simulink model "aircraftRamAirTurbineAssembly_MultiDomain"  (Simulink 7.9)
settings: Solver=ode23tb  StartTime=0.0  StopTime=6  FixedStep=Ts  MaxStep=50e-6  RelTol=1e-4
PreLoadFcn:
  | % PARAMETERS FOR HYDRAULIC CYLINDER
  | RO = 0.1;
  | t = 0.005;
  | h = 2.5;
  | lic = -1.1;
  | rho = 1000;
  | 
  | APist = pi*(RO - 2*t)*(RO - 2*t);
  | ROO = RO;
  | RIO = RO - t;
  | ROI = RO-t;
  | RII = RO- 2*t;
  | h_seg = h/2;
  | 
  | ro = ROO;
  | ri = RIO;
  | h = h_seg;
  | rho = rho;
  | rot_oc = [0 0 165];
  | 
  | mass_OC = rho*pi*(ro*ro-ri*ri)*h;
  | inertia_OC = mass_OC*([(3*ro*ro + h*h) 0 0;0 6*ro*ro 0;0 0 (3*ro*ro + h*h)]-[(3*ri*ri + h*h) 0 0;0 6*ri*ri 0;0 0 (3*ri*ri + h*h)])/12;
  | 
  | ro = ROI;
  | ri = RII;
  | h = h_seg;
  | rho = rho;
  | rot_ic = [0 0 0];
  | 
  | mass_IC = rho*pi*(ro*ro-ri*ri)*h;
  | inertia_IC = mass_IC*([(3*ro*ro + h*h) 0 0;0 6*ro*ro 0;0 0 (3*ro*ro + h*h)]-[(3*ri*ri + h*h) 0 0;0 6*ri*ri 0;0 0 (3*ri*ri + h*h)])/12;
  | 
  | a = 0.1;
  | b = 2;
  | c = 0.05;
  | rho = 1000;
  | theta = 180;
  | 
  | mass_Link = rho*a*b*c;
  | inertia_Link = rho*a*b*c*[(b^2+c^2) 0 0; 0 (a^2+c^2) 0; 0 0 (a^2+b^2)]/12;
  | 
  | Actuator_Attach_Pt = [0 -0.2 0];
  | Actuator_Wing_Pt = [-0.5 0 0];
  | Outer_Cylinder_Length = 0.35;
  | Inner_Cylinder_Length = 0.25;
  | 
  | Outer_Cyl_Axis = Actuator_Wing_Pt - Actuator_Attach_Pt;
  | %Outer_Cyl_Axis = Outer_Cyl_Axis/(sqrt(sum(Outer_Cyl_Axis.*Outer_Cyl_Axis)));
  | 
  | %Actuator_Angle = atan(Outer_Cyl_Axis(2)/Outer_Cyl_Axis(1))*180/pi;
  | Actuator_Angle = -10;
  | Outer_Cyl_CS2 = Outer_Cyl_Axis*Outer_Cylinder_Length;
  | 
  | Cylinder_Overlap = 0.05 ;
  | 
  | Signal_Times = linspace(0,0.5,11);
  | Signal_Values = [0 1 1 0 0 -1 -1 0 0 0 0];
  | 
  | Airfoil_Length = 1;
  | Airfoil_Thickness_1 = 0.25;
  | Airfoil_Thickness_2 = 0.2;
  | Airfoil_Offset_1=0.15;
  | Airfoil_Offset_2=-0.13;
  | Airfoil_Nose_Length = 0.10;
  | 
  | Wind_Offset = 0.7;
  | 
  | Ka = 1*1e-1;
  | Kb = 2500;
  | 
  | Ka_Final = 0.1791;
  | Kb_Final = 343.75;
  | Kp = 0.3;Ki=0.3;
  | Ts=25e-6;
InitFcn:
  | Ts_pwm=5e-6;
  | or_width = 24.5;
  | x0_PA = 0.01;
  | x0_PB = 0.01;
  | x0_AT = 0.01;
  | x0_BT = 0.01;
  | rad_clearance = 5e-2;
  | 
  | % PARAMETERS FOR HYDRAULIC CYLINDER
  | RO = 0.1;
  | t = 0.005;
  | h = 2.5;
  | lic = -1.1;
  | rho = 1000;
  | 
  | APist = pi*(RO - 2*t)*(RO - 2*t);
  | ROO = RO;
  | RIO = RO - t;
  | ROI = RO-t;
  | RII = RO- 2*t;
  | h_seg = h/2;
  | 
  | ro = ROO;
  | ri = RIO;
  | h = h_seg;
  | rho = rho;
  | rot_oc = [0 0 165];
  | 
  | mass_OC = rho*pi*(ro*ro-ri*ri)*h;
  | inertia_OC = mass_OC*([(3*ro*ro + h*h) 0 0;0 6*ro*ro 0;0 0 (3*ro*ro + h*h)]-[(3*ri*ri + h*h) 0 0;0 6*ri*ri 0;0 0 (3*ri*ri + h*h)])/12;
  | 
  | ro = ROI;
  | ri = RII;
  | h = h_seg;
  | rho = rho;
  | rot_ic = [0 0 0];
  | 
  | mass_IC = rho*pi*(ro*ro-ri*ri)*h;
  | inertia_IC = mass_IC*([(3*ro*ro + h*h) 0 0;0 6*ro*ro 0;0 0 (3*ro*ro + h*h)]-[(3*ri*ri + h*h) 0 0;0 6*ri*ri 0;0 0 (3*ri*ri + h*h)])/12;
  | 
  | a = 0.1;
  | b = 2;
  | c = 0.05;
  | rho = 1000;
  | theta = 180;
  | 
  | mass_Link = rho*a*b*c;
  | inertia_Link = rho*a*b*c*[(b^2+c^2) 0 0; 0 (a^2+c^2) 0; 0 0 (a^2+b^2)]/12;
  | 
  | Actuator_Attach_Pt = [0 -0.2 0];
  | Actuator_Wing_Pt = [-0.5 0 0];
  | Outer_Cylinder_Length = 0.35;
  | Inner_Cylinder_Length = 0.25;
  | 
  | Outer_Cyl_Axis = Actuator_Wing_Pt - Actuator_Attach_Pt;
  | %Outer_Cyl_Axis = Outer_Cyl_Axis/(sqrt(sum(Outer_Cyl_Axis.*Outer_Cyl_Axis)));
  | 
  | %Actuator_Angle = atan(Outer_Cyl_Axis(2)/Outer_Cyl_Axis(1))*180/pi;
  | Actuator_Angle = -10;
  | Outer_Cyl_CS2 = Outer_Cyl_Axis*Outer_Cylinder_Length;
  | 
  | Cylinder_Overlap = 0.05 ;
  | 
  | Signal_Times = linspace(0,0.5,11);
  | Signal_Values = [0 1 1 0 0 -1 -1 0 0 0 0];
  | 
  | Airfoil_Length = 1;
  | Airfoil_Thickness_1 = 0.25;
  | Airfoil_Thickness_2 = 0.2;
  | Airfoil_Offset_1=0.15;
  | Airfoil_Offset_2=-0.13;
  | Airfoil_Nose_Length = 0.10;
  | 
  | Wind_Offset = 0.7;
  | 
  | Ka = 1*1e-1;
  | Kb = 2500;
  | 
  | Ka_Final = 0.1791;
  | Kb_Final = 343.75;
  | Kp = 0.3;Ki=0.3;
  | Ts=25e-6;
undefined symbols (not defined in the file or in its folder): D1, Delta
libraries: fl_lib x36, nesl_utility x17, mblibv1 x16, sh_lib x15, powerlib x10, powerlib_extras x6, simulink x1, DRlib x1
(part 1 of 2)
Description:
  | Copyright 2008-2009 The MathWorks(TM), Inc.
settings Model: FPTRunName=Active  Creator=rhassan  LastModifiedBy=PMercier
settings DataIOCC: LimitDataPoints=off  SaveOutput=off  SignalLogging=off  SaveTime=off
settings OptimizationCC: InitFltsAndDblsToZero=on
settings DebuggingCC: SaveWithParameterizedLinksMsg=none  FcnCallInpInsideContextMsg=Use local settings  StrictBusMsg=Warning
settings GRTTargetCC: TargetFcnLib=ansi_tfl_tmw.mat  CombineOutputUpdateFcns=off  GRTInterface=on
settings SimscapeCC: ExplicitSolverDiagnosticOptions=none
settings ConfigurationSet: Description=SimMechanics 2G

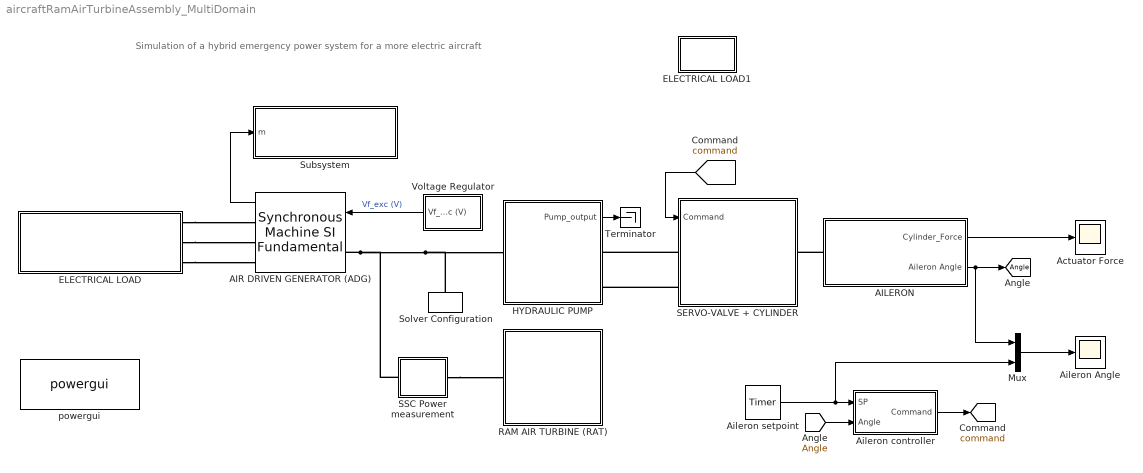
== system aircraftRamAirTurbineAssembly_MultiDomain ==
  note: Simulation of a hybrid emergency power system for a more electric aircraft
  AILERON : Subsystem  RequirementInfo={'other' 'Aileron_Requirements.doc' '@path_module' 'true' 'Mechanical System Requirements ' '' } %GIDa_ce3fe074_9f1c_4d4f_9959_ef64db326e2e
      mask Display: image(imread('Aileron_Diagram.JPG'));
  AIR DRIVEN GENERATOR (ADG) : powerlib/Machines/Synchronous Machine SI Fundamental  PresetModel=No  MechanicalLoad=Mechanical rotational port  ShowDetailedParameters=on  RotorType=Salient-pole  NominalParameters=[1.5e+004 200 400 50]  Stator=[0.114 .18e-3 1.82e-3 1.6e-3]  Field=[0.015 0.255e-3]  Dampers2=[ 0.0664, 1.387e-3, 0.0292, 6.896e-4, 7.907e-3, 2.477e-3]  Dampers1=[0.118 0.650e-3 .110 0.06e-3]  Mechanical=[0.0026 0.0013 3]  PolePairs=3  InitialConditions="[0 0 0 0 0 0 0 0  0]"  SetSaturation=off  Saturation=[695.64,774.7,917.5,1001.6,1082.2,1175.9,1293.6,1430.2,1583.7;9660,10623,12243,13063,13757,14437,15180,15890,16567]  DisplayVfd=off  Units=SI fundamental parameters  LoadFlowParameters=[1,0,0,0,0]  TsPowergui=0  TsBlock=Ts  IterativeModel=Forward Euler  BusType=PV  Pref=0  Qref=0  Qmin=-inf  Qmax=inf  PLF=0  QLF=0
  Actuator Force : Scope
      settings: TimeRange=5  YMin=-200.413  YMax=-200.406  SaveName=Aileron_EH_Force_DATA
  Aileron Angle : Scope
      settings: TimeRange=6  YMin=-20  YMax=15  SaveName=Aileron_EH_Angle_DATA
  Aileron setpoint : powerlib_extras/Control  Blocks/Timer  t=[ 0 1 3]  e="[0  10 -15]"
  Aileron controller : Subsystem
  ELECTRICAL LOAD : Subsystem
      mask Display: image(imread('res.jpg','jpg'))
  ELECTRICAL LOAD1 : Subsystem
      settings: OpenFcn=showdemo('aircraftRamAirTurbineAssembly_MultiDomain')
      mask Display: disp('HELP')
  HYDRAULIC PUMP : Subsystem
      mask Display: image(imread('power_Hydraulic_Pump_Pump.jpg','jpg'))
  Mux : Mux  Inputs=2
  RAM AIR TURBINE (RAT) : Subsystem
      mask Display:
      | plot(0,0,118,100)
      | plot([56 62],[4 4],[56 57],[4 52],[62 61],[4 52])
      | plot([57 59 61],[52 52.5 52])
      | plot([61 61.5 62 63 63],[52 52.2 52.5 54 56])
      | plot([63 59 57.6 57.3 56 55],[56 58 57.8 55.6 54.2 54])
      | plot([55 57],[54 52],[57.3 63],[55.6 54])
      | plot([57.6 57 55 54.7 60 81],[57.6 57.3 58 59.4 64 82])
      | plot([81 83 84 84.2 83 81],[82 83.6 83.4 83 80.8 78.7])
      | plot([81 60.5 57.6],[78.7 60 57.6])
      | plot([54.7 53 51 51.3 52.5],[59.4 58.8 58 56 55])
      | plot([52.5 53.7 54.5 55],[55 54.9 54.6 54])
      | plot([51 47 35 33 32 33 35],[58 59 66 67.7 68.5 68.4 68])
      | plot([35 45 52 53 53.7],[68 64 61 60 59.2])
      | plot([52.5 51 50.8 51.5 55],[55 26 21 26 54])
  SERVO-VALVE + CYLINDER : Subsystem
      mask Display: image(imread('servovalve.jpg', 'jpg'))
  SSC Power measurement : Subsystem
  Solver Configuration : nesl_utility/Solver Configuration  PhysicalDomain=network_engine_domain  LeftPortType=input  RightPortType=generic  SubClassName=solver  UseCustomDae=off  DoDC=off  ResidualTolerance=1e-9  UseLocalSolver=on  LocalSolverChoice=NE_BACKWARD_EULER_ADVANCER  LocalSolverSampleTime=Ts  DoFixedCost=on  MaxNonlinIter=3  MaxModeIter=2  LinearAlgebra=Sparse  Accelerate=off  Profile=off  UseLocalSampling=off  DelaysMemoryBudget=1024
  Subsystem : Subsystem
      mask Display: fprintf('Measurements','Bold')
  Terminator : Terminator
  Voltage Regulator : Subsystem
  powergui : powerlib/powergui  SimulationMode=Discrete  SolverType=Tustin  SampleTime=Ts  frequency=60  SPID=off  DisableSnubberDevices=off  DisableRonSwitches=off  DisableVfSwitches=off  SwTol=0  Interpol=off  DisplayEquations=off  FunctionMessages=off  frequencyindice=0  Pbase=100e6  ErrMax=1e-4  Iterations=50  UnitsV=kV  UnitsW=MW  echomessages=off  HookPort=off  EnableUseOfTLC=off  x0status=blocks  RestoreLinks=warning  ResistiveCurrentMeasurement=off  Frange=[0:2:500]  Ylog=off  Xlog=on  ShowGrid=off  save=off  variable=ZData  structure=Ctrl_Sig  ZoomFFT=on  StartTime=0.0  cycles=1  DisplayStyle=1  fundamental=60  FreqAxis=off  MaxFrequency=1000  frequencyindicesteady=1  RmsSteady=1  display=off  Ts=0  methode=off
  tag scope: Angle=global, command=global
  wires:
  Voltage Regulator/1(Vf_exc (V)) -> AIR DRIVEN GENERATOR (ADG)/1  "Vf_exc (V)"
  AILERON/1(Cylinder_Force) -> Actuator Force/1
  AILERON/2(Aileron Angle) -> [Angle], Mux/1
  [Angle] -> Aileron controller/2(Angle)
  Aileron controller/1(Command) -> [command]
  [command] -> SERVO-VALVE + CYLINDER/1(Command)
  Aileron setpoint/1 -> Aileron controller/1(SP), Mux/2
  Mux/1 -> Aileron Angle/1
  HYDRAULIC PUMP/1(Pump_output) -> Terminator/1
  AIR DRIVEN GENERATOR (ADG)/1 -> Subsystem/1(m)
  connections:
  AIR DRIVEN GENERATOR (ADG)/LConn1 -- Solver Configuration/RConn1 -- HYDRAULIC PUMP/LConn1 -- SSC Power measurement/RConn1
  SERVO-VALVE + CYLINDER/LConn2 -- HYDRAULIC PUMP/RConn2
  SERVO-VALVE + CYLINDER/LConn1 -- HYDRAULIC PUMP/RConn1
  AILERON/LConn1 -- SERVO-VALVE + CYLINDER/RConn1
  SSC Power measurement/LConn1 -- RAM AIR TURBINE (RAT)/LConn1
  ELECTRICAL LOAD/RConn1 -- AIR DRIVEN GENERATOR (ADG)/RConn1
  ELECTRICAL LOAD/RConn2 -- AIR DRIVEN GENERATOR (ADG)/RConn2
  ELECTRICAL LOAD/RConn3 -- AIR DRIVEN GENERATOR (ADG)/RConn3

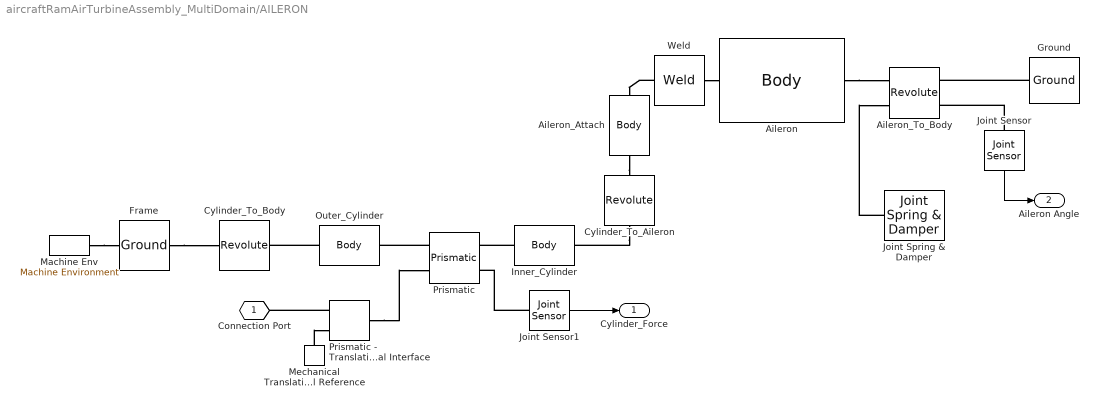
== system aircraftRamAirTurbineAssembly_MultiDomain/AILERON ==
  Aileron : mblibv1/Bodies/Body  LConnTagsString=CS3  RConnTagsString=CS1  UpdateFromCAD=off  DialogClass=MechanicalBodyBlock  Mass=mass_Link  MassUnits=kg  InertiaUnits=kg*m^2  Inertia=inertia_Link  Shape=Cylinder  ShapeDims=[1 1]  ShapeUnits=m  ShapeUse=false  Density=1  DensityUnits=kg/m^3  DensityUse=false  GraphicsMode=MACHINE_DEFAULT  BodyColorSelMode=MACHINE_DEFAULT  BodyColor=[0.5 0.5 0.5]  AttachedToCS=CG  CG=Left$CG$[-Airfoil_Length/5 0 0]$CS1$CS1$m$[0 0 0]$Euler X-Y-Z$deg$CS1$false$none  WorkingFrames=Right$CS1$[0 0 0]$ADJOINING$ADJOINING$m$[0 0 theta]$Euler X-Y-Z$deg$ADJOINING$true$none#Right$CS2$[-Airfoil_Length 0 1]$CS1$CS1$m$[0 0 0]$Euler X-Y-Z$deg$CS1$false$none#Right$CS16$[-Airfoil_Length 0 -1]$CS1$CS1$m$[0 0 0]$Euler X-Y-Z$deg$CS1$false$none#Right$CS9$[-Airfoil_Length*Wind_Offset 0 1]$CS1$CS1$m$[0 0 0]$Euler X-Y-Z$deg$CS1$false$none#Right$CS15$[-Airfoil_Length*Wind_Offset 0 -1]$CS1$CS1$m$[0 0 0]$Euler X-Y-Z$deg$CS1$false$none#Right$CS8$[Airfoil_Nose_Length 0 1]$CS1$CS1$m$[0 0 0]$Euler X-Y-Z$deg$CS1$false$none#Right$CS14$[Airfoil_Nose_Length 0 -1]$CS1$CS1$m$[0 0 0]$Euler X-Y-Z$deg$CS1$false$none#Left$CS4$[-Airfoil_Length*Airfoil_Offset_1 Airfoil_Thickness_1/2 1]$CG$CG$m$[0 0 0]$Euler X-Y-Z$deg$CG$false$none#Left$CS10$[-Airfoil_Length*Airfoil_Offset_1 Airfoil_Thickness_1/2 -1]$CG$CG$m$[0 0 0]$Euler X-Y-Z$deg$CG$false$none#Left$CS5$[-Airfoil_Length*Airfoil_Offset_1 -Airfoil_Thickness_1/2 1]$CG$CG$m$[0 0 0]$Euler X-Y-Z$deg$CG$false$none#Left$CS11$[-Airfoil_Length*Airfoil_Offset_1 -Airfoil_Thickness_1/2 -1]$CG$CG$m$[0 0 0]$Euler X-Y-Z$deg$CG$false$none#Left$CS6$[-Airfoil_Length*Airfoil_Offset_2 -Airfoil_Thickness_2/2 1]$CG$CG$m$[0 0 0]$Euler X-Y-Z$deg$CG$false$none#Left$CS12$[-Airfoil_Length*Airfoil_Offset_2 -Airfoil_Thickness_2/2 -1]$CG$CG$m$[0 0 0]$Euler X-Y-Z$deg$CG$false$none#Left$CS7$[-Airfoil_Length*Airfoil_Offset_2 Airfoil_Thickness_2/2 1]$CG$CG$m$[0 0 0]$Euler X-Y-Z$deg$CG$false$none#Left$CS13$[-Airfoil_Length*Airfoil_Offset_2 Airfoil_Thickness_2/2 -1]$CG$CG$m$[0 0 0]$Euler X-Y-Z$deg$CG$false$none#Left$CS3$[0 0 0]$CS1$CS1$m$[0 0 0]$Euler X-Y-Z$deg$CG$true$none  CGPos=[-Airfoil_Length/5 0 0]  CGRot=[0 0 0]  CS0Pos=[]  CS0Rot=[]  CS1Pos=[0 0 0]  CS1Rot=[0 0 theta]  CS2Pos=[-Airfoil_Length 0 1]  CS2Rot=[0 0 0]  CS3Pos=[0 0 0]  CS3Rot=[0 0 0]  CS4Pos=[-Airfoil_Length*Airfoil_Offset_1 Airfoil_Thickness_1/2 1]  CS4Rot=[0 0 0]  CS5Pos=[-Airfoil_Length*Airfoil_Offset_1 -Airfoil_Thickness_1/2 1]  CS5Rot=[0 0 0]  CS6Pos=[-Airfoil_Length*Airfoil_Offset_2 -Airfoil_Thickness_2/2 1]  CS6Rot=[0 0 0]  CS7Pos=[-Airfoil_Length*Airfoil_Offset_2 Airfoil_Thickness_2/2 1]  CS7Rot=[0 0 0]  CS8Pos=[Airfoil_Nose_Length 0 1]  CS8Rot=[0 0 0]  CS9Pos=[-Airfoil_Length*Wind_Offset 0 1]  CS9Rot=[0 0 0]  CS10Pos=[-Airfoil_Length*Airfoil_Offset_1 Airfoil_Thickness_1/2 -1]  CS10Rot=[0 0 0]  CS11Pos=[-Airfoil_Length*Airfoil_Offset_1 -Airfoil_Thickness_1/2 -1]  CS11Rot=[0 0 0]  CS12Pos=[-Airfoil_Length*Airfoil_Offset_2 -Airfoil_Thickness_2/2 -1]  CS12Rot=[0 0 0]  CS13Pos=[-Airfoil_Length*Airfoil_Offset_2 Airfoil_Thickness_2/2 -1]  CS13Rot=[0 0 0]  CS14Pos=[Airfoil_Nose_Length 0 -1]  CS14Rot=[0 0 0]  CS15Pos=[-Airfoil_Length*Wind_Offset 0 -1]  CS15Rot=[0 0 0]  CS16Pos=[-Airfoil_Length 0 -1]  CS16Rot=[0 0 0]  CS17Pos=[]  CS17Rot=[]  CS18Pos=[]  CS18Rot=[]  CS19Pos=[]  CS19Rot=[]  CS20Pos=[]  CS20Rot=[]
  Aileron_Attach : mblibv1/Bodies/Body  LConnTagsString=CS1  RConnTagsString=CS2  UpdateFromCAD=off  DialogClass=MechanicalBodyBlock  Mass=1  MassUnits=kg  InertiaUnits=kg*m^2  Inertia=eye(3)  Shape=Cylinder  ShapeDims=[1 1]  ShapeUnits=m  ShapeUse=false  Density=1  DensityUnits=kg/m^3  DensityUse=false  GraphicsMode=MACHINE_DEFAULT  BodyColorSelMode=MACHINE_DEFAULT  BodyColor=[0.5 0.5 0.5]  AttachedToCS=CG  CG=Left$CG$[0 0 0]$CS2$CS2$m$[0 0 0]$Euler X-Y-Z$deg$WORLD$false$none  WorkingFrames=Left$CS1$[0 0 0]$Adjoining$Adjoining$m$[0 0 0]$Euler X-Y-Z$deg$WORLD$true$none#Right$CS2$[0 0 0]$Adjoining$Adjoining$m$[0 0 0]$Euler X-Y-Z$deg$WORLD$true$none  CGPos=[0 0 0]  CGRot=[0 0 0]  CS0Pos=[]  CS0Rot=[]  CS1Pos=[0 0 0]  CS1Rot=[0 0 0]  CS2Pos=[0 0 0]  CS2Rot=[0 0 0]  CS3Pos=[]  CS3Rot=[]  CS4Pos=[]  CS4Rot=[]  CS5Pos=[]  CS5Rot=[]  CS6Pos=[]  CS6Rot=[]  CS7Pos=[]  CS7Rot=[]  CS8Pos=[]  CS8Rot=[]  CS9Pos=[]  CS9Rot=[]  CS10Pos=[]  CS10Rot=[]  CS11Pos=[]  CS11Rot=[]  CS12Pos=[]  CS12Rot=[]  CS13Pos=[]  CS13Rot=[]  CS14Pos=[]  CS14Rot=[]  CS15Pos=[]  CS15Rot=[]  CS16Pos=[]  CS16Rot=[]  CS17Pos=[]  CS17Rot=[]  CS18Pos=[]  CS18Rot=[]  CS19Pos=[]  CS19Rot=[]  CS20Pos=[]  CS20Rot=[]
  Aileron_To_Body : mblibv1/Joints/Revolute  LConnTagsString=__newl0|SA1  RConnTagsString=__newr0|SA1  UpdateFromCAD=off  NumSAPorts=2  CutJoint=off  MarkAsCut=off  Primitives=revolute  PrimitiveProps=R1$World$[0 0 1]$revolute  DialogClass=JointBlock  R1Axis=[0 0 1]
  Cylinder_To_Aileron : mblibv1/Joints/Revolute  LConnTagsString=__newl0  RConnTagsString=__newr0  UpdateFromCAD=off  NumSAPorts=0  CutJoint=off  MarkAsCut=off  Primitives=revolute  PrimitiveProps=R1$World$[0 0 1]$revolute  DialogClass=JointBlock  R1Axis=[0 0 1]
  Cylinder_To_Body : mblibv1/Joints/Revolute  LConnTagsString=__newl0  RConnTagsString=__newr0  UpdateFromCAD=off  NumSAPorts=0  CutJoint=off  MarkAsCut=off  Primitives=revolute  PrimitiveProps=R1$World$[0 0 1]$revolute  DialogClass=JointBlock  R1Axis=[0 0 1]
  Frame : mblibv1/Bodies/Ground  UpdateFromCAD=off  LeftPortType=env  RightPortType=workingframe  PhysicalDomain=Mechanical  DialogClass=GroundBlock  CoordPosition=Actuator_Wing_Pt  CoordPositionUnits=m  StateVectorMgrId=1  MachineId=[2 0]  ShowEnvPort=on
  Ground : mblibv1/Bodies/Ground  UpdateFromCAD=off  LeftPortType=env  RightPortType=workingframe  PhysicalDomain=Mechanical  DialogClass=GroundBlock  CoordPosition=[0 0 0]  CoordPositionUnits=m  StateVectorMgrId=-1  MachineId=[0 0]  ShowEnvPort=off
  Inner_Cylinder : mblibv1/Bodies/Body  LConnTagsString=CS1  RConnTagsString=CS2  UpdateFromCAD=off  DialogClass=MechanicalBodyBlock  Mass=mass_IC  MassUnits=kg  InertiaUnits=kg*m^2  Inertia=inertia_IC  Shape=Cylinder  ShapeDims=[1 1]  ShapeUnits=m  ShapeUse=false  Density=1  DensityUnits=kg/m^3  DensityUse=false  GraphicsMode=MACHINE_DEFAULT  BodyColorSelMode=MACHINE_DEFAULT  BodyColor=[0.5 0.5 0.5]  AttachedToCS=CG  CG=Left$CG$[Inner_Cylinder_Length/2 0 0]$CS1$CS1$m$[0 0 0]$Euler X-Y-Z$deg$CS1$false$none  WorkingFrames=Left$CS1$[-Cylinder_Overlap 0 0]$ADJOINING$ADJOINING$m$[0 0 0]$Euler X-Y-Z$deg$ADJOINING$true$none#Right$CS2$[Inner_Cylinder_Length 0 0]$CS1$CS1$m$[0 0 0]$Euler X-Y-Z$deg$CG$true$none  CGPos=[Inner_Cylinder_Length/2 0 0]  CGRot=[0 0 0]  CS0Pos=[]  CS0Rot=[]  CS1Pos=[-Cylinder_Overlap 0 0]  CS1Rot=[0 0 0]  CS2Pos=[Inner_Cylinder_Length 0 0]  CS2Rot=[0 0 0]  CS3Pos=[]  CS3Rot=[]  CS4Pos=[]  CS4Rot=[]  CS5Pos=[]  CS5Rot=[]  CS6Pos=[]  CS6Rot=[]  CS7Pos=[]  CS7Rot=[]  CS8Pos=[]  CS8Rot=[]  CS9Pos=[]  CS9Rot=[]  CS10Pos=[]  CS10Rot=[]  CS11Pos=[]  CS11Rot=[]  CS12Pos=[]  CS12Rot=[]  CS13Pos=[]  CS13Rot=[]  CS14Pos=[]  CS14Rot=[]  CS15Pos=[]  CS15Rot=[]  CS16Pos=[]  CS16Rot=[]  CS17Pos=[]  CS17Rot=[]  CS18Pos=[]  CS18Rot=[]  CS19Pos=[]  CS19Rot=[]  CS20Pos=[]  CS20Rot=[]
  Joint Sensor : mblibv1/Sensors &  Actuators/Joint Sensor  UpdateFromCAD=off  PhysicalDomain=Mechanical  PortType=blob  Muxed=on  Pose=off  Angle=on  AngleUnits=deg  ArcVelocity=off  ArcVelocityUnits=deg/s  ArcAcceleration=off  ArcAccelerationUnits=deg/s^2  CoordPosition=on  CoordPositionUnits=m  Velocity=off  VelocityUnits=m/s  Acceleration=off  AccelerationUnits=m/s^2  Quaternion=on  QuaternionDT=off  QuaternionDDT=off  QuaternionUnits=off  OutputVector=[1]  ActiveIO=on  Width=1  DialogClass=MechanicalSensorBlock  Primitive=R1  Force=off  ForceUnits=N  Torque=off  TorqueUnits=N*m  ReferenceFrame=Absolute (World)  ReactionSensedSide=Base  ReactionReferenceFrame=Absolute (World)  ReactionForce=off  ReactionForceUnits=N  ReactionMoment=off  ReactionMomentUnits=N*m
  Joint Sensor1 : mblibv1/Sensors &  Actuators/Joint Sensor  UpdateFromCAD=off  PhysicalDomain=Mechanical  PortType=blob  Muxed=on  Pose=off  Angle=on  AngleUnits=deg  ArcVelocity=off  ArcVelocityUnits=deg/s  ArcAcceleration=off  ArcAccelerationUnits=deg/s^2  CoordPosition=off  CoordPositionUnits=m  Velocity=off  VelocityUnits=m/s  Acceleration=off  AccelerationUnits=m/s^2  Quaternion=on  QuaternionDT=off  QuaternionDDT=off  QuaternionUnits=off  OutputVector=[1]  ActiveIO=on  Width=1  DialogClass=MechanicalSensorBlock  Primitive=P1  Force=on  ForceUnits=N  Torque=off  TorqueUnits=N*m  ReferenceFrame=Absolute (World)  ReactionSensedSide=Base  ReactionReferenceFrame=Absolute (World)  ReactionForce=off  ReactionForceUnits=N  ReactionMoment=off  ReactionMomentUnits=N*m
  Joint Spring & Damper : mblibv1/Force  Elements/Joint Spring & Damper  UpdateFromCAD=off  DialogClass=JointSpringDamper  JFEParameters=P1$false$0$0$0$m$m/s$N$deg$deg/s$N*m#P2$false$0$0$0$m$m/s$N$deg$deg/s$N*m#P3$false$0$0$0$m$m/s$N$deg$deg/s$N*m#R1$true$0$10$0$m$m/s$N$deg$deg/s$N*m#R2$false$0$0$0$m$m/s$N$deg$deg/s$N*m#R3$false$0$0$0$m$m/s$N$deg$deg/s$N*m#S$false$0$0$0$m$m/s$N$deg$deg/s$N*m
  Machine Env : mblibv1/Bodies/Machine Environment  Tag=Factory ground  PortType=env  PhysicalDomain=Mechanical  DialogTemplateClass=MECH.MachineEnvironment  SyncWhenCopied=off  Gravity=[0 -9.81 0]  GravityUnits=m/s^2  GravityAsSignal=off  Dimensionality=Auto-detect  AnalysisType=Forward dynamics  LinearAssemblyTolerance=1e-3  LinearAssemblyToleranceUnits=m  AngularAssemblyTolerance=1e-3  AngularAssemblyToleranceUnits=rad  ConstraintSolverType=Stabilizing  ConstraintRelTolerance=1e-4  ConstraintAbsTolerance=1e-4  UseRobustSingularityHandling=off  RedundancyAnalysisToleranceType=Automatically select tolerance  RedundancyAnalysisTolerance=1e-14  StatePerturbationType=Fixed  PerturbationSize=1e-5  VisualizeMachine=off  BodyVisualizationType=Convex hull from body CS locations  BodyColorSelMode=Use model default  DefaultBodyColor=[1 0 0]
  Mechanical Translational Reference : fl_lib/Mechanical/Translational Elements/Mechanical Translational Reference  f_Log=off  LocalVarNames=|f  LocalVarDescs=|f  LocalVarLogging=[]
  Outer_Cylinder : mblibv1/Bodies/Body  LConnTagsString=CS1  RConnTagsString=CS2  UpdateFromCAD=off  DialogClass=MechanicalBodyBlock  Mass=mass_OC  MassUnits=kg  InertiaUnits=kg*m^2  Inertia=inertia_OC  Shape=Cylinder  ShapeDims=[1 1]  ShapeUnits=m  ShapeUse=false  Density=1  DensityUnits=kg/m^3  DensityUse=false  GraphicsMode=MACHINE_DEFAULT  BodyColorSelMode=MACHINE_DEFAULT  BodyColor=[0.5 0.5 0.5]  AttachedToCS=CG  CG=Left$CG$[Outer_Cylinder_Length/2 0 0]$CS1$CS1$m$[0 0 0]$Euler X-Y-Z$deg$CS1$false$none  WorkingFrames=Left$CS1$[0 0 0]$ADJOINING$ADJOINING$m$[0 0 Actuator_Angle]$Euler X-Y-Z$deg$Adjoining$true$none#Right$CS2$[Outer_Cylinder_Length 0 0]$CS1$CS1$m$[0 0 0]$Euler X-Y-Z$deg$CG$true$none  CGPos=[Outer_Cylinder_Length/2 0 0]  CGRot=[0 0 0]  CS0Pos=[]  CS0Rot=[]  CS1Pos=[0 0 0]  CS1Rot=[0 0 Actuator_Angle]  CS2Pos=[Outer_Cylinder_Length 0 0]  CS2Rot=[0 0 0]  CS3Pos=[]  CS3Rot=[]  CS4Pos=[]  CS4Rot=[]  CS5Pos=[]  CS5Rot=[]  CS6Pos=[]  CS6Rot=[]  CS7Pos=[]  CS7Rot=[]  CS8Pos=[]  CS8Rot=[]  CS9Pos=[]  CS9Rot=[]  CS10Pos=[]  CS10Rot=[]  CS11Pos=[]  CS11Rot=[]  CS12Pos=[]  CS12Rot=[]  CS13Pos=[]  CS13Rot=[]  CS14Pos=[]  CS14Rot=[]  CS15Pos=[]  CS15Rot=[]  CS16Pos=[]  CS16Rot=[]  CS17Pos=[]  CS17Rot=[]  CS18Pos=[]  CS18Rot=[]  CS19Pos=[]  CS19Rot=[]  CS20Pos=[]  CS20Rot=[]
  Prismatic : mblibv1/Joints/Prismatic  LConnTagsString=__newl0|SA1  RConnTagsString=__newr0|SA1  UpdateFromCAD=off  NumSAPorts=2  CutJoint=off  MarkAsCut=off  Primitives=prismatic  PrimitiveProps=P1$Base$[-1 0 0] $prismatic  DialogClass=JointBlock  P1Axis=[-1 0 0]
  Prismatic - Translational Interface : mblibv1/Interface  Elements/Prismatic - Translational Interface  UpdateFromCAD=off  DialogClass=PrismaticTranslationalInterface  Primitive=P1
  Weld : mblibv1/Joints/Weld  LConnTagsString=__newl0  RConnTagsString=__newr0  UpdateFromCAD=off  NumSAPorts=0  CutJoint=off  MarkAsCut=off  Primitives=weld  PrimitiveProps=W$World$[0 0 0]$weld  DialogClass=JointBlock  WAxis=[0 0 0]
  Connection Port : PMIOPort  Port=1  Side=Left
  Cylinder_Force : Outport
  Aileron Angle : Outport  Port=2
  wires:
  Joint Sensor1/1 -> Cylinder_Force/1
  Joint Sensor/1 -> Aileron Angle/1
  connections:
  Joint Sensor1/LConn1 -- Prismatic/RConn2
  Machine Env/RConn1 -- Frame/LConn1
  Prismatic/LConn1 -- Outer_Cylinder/RConn1
  Inner_Cylinder/LConn1 -- Prismatic/RConn1
  Outer_Cylinder/LConn1 -- Cylinder_To_Body/RConn1
  Frame/RConn1 -- Cylinder_To_Body/LConn1
  Cylinder_To_Aileron/LConn1 -- Inner_Cylinder/RConn1
  Joint Sensor/LConn1 -- Aileron_To_Body/LConn2
  Ground/RConn1 -- Aileron_To_Body/LConn1
  Weld/RConn1 -- Aileron_Attach/RConn1
  Aileron_Attach/LConn1 -- Cylinder_To_Aileron/RConn1
  Aileron/RConn1 -- Aileron_To_Body/RConn1
  Weld/LConn1 -- Aileron/LConn1
  Joint Spring & Damper/LConn1 -- Aileron_To_Body/RConn2
  Mechanical Translational Reference/LConn1 -- Prismatic - Translational Interface/LConn2
  Prismatic - Translational Interface/LConn1 -- Connection Port/RConn1
  Prismatic - Translational Interface/RConn1 -- Prismatic/LConn2

== system aircraftRamAirTurbineAssembly_MultiDomain/Aileron controller ==
  SP : Inport
  Angle : Inport  Port=2
  Add : Sum  Inputs=|+-
  PID Controller : simulink/Continuous/PID Controller  Controller=PD  TimeDomain=Continuous-time  SampleTime=1  IntegratorMethod=Forward Euler  FilterMethod=Forward Euler  Form=Parallel  P=0.01  I=0.0001  D=0.001  N=1000  InitialConditionSource=internal  InitialConditionForIntegrator=0  InitialConditionForFilter=0  ExternalReset=none  LimitOutput=off  UpperSaturationLimit=inf  LowerSaturationLimit=-inf  LinearizeAsGain=off  AntiWindupMode=none  Kb=1  TrackingMode=off  Kt=1  PParamMin=[]  PParamMax=[]  IParamMin=[]  IParamMax=[]  DParamMin=[]  DParamMax=[]  NParamMin=[]  NParamMax=[]  KbParamMin=[]  KbParamMax=[]  KtParamMin=[]  KtParamMax=[]  POutMin=[]  POutMax=[]  IOutMin=[]  IOutMax=[]  DOutMin=[]  DOutMax=[]  NOutMin=[]  NOutMax=[]  KbOutMin=[]  KbOutMax=[]  KtOutMin=[]  KtOutMax=[]  IntegratorOutMin=[]  IntegratorOutMax=[]  FilterOutMin=[]  FilterOutMax=[]  SumOutMin=[]  SumOutMax=[]  SumI1OutMin=[]  SumI1OutMax=[]  SumI2OutMin=[]  SumI2OutMax=[]  SumI3OutMin=[]  SumI3OutMax=[]  SumDOutMin=[]  SumDOutMax=[]  SaturationOutMin=[]  SaturationOutMax=[]  IntegratorContinuousStateAttributes=''  IntegratorStateMustResolveToSignalObject=off  IntegratorRTWStateStorageClass=Auto  FilterContinuousStateAttributes=''  FilterStateMustResolveToSignalObject=off  FilterRTWStateStorageClass=Auto
  Command : Outport
  wires:
  Add/1 -> PID Controller/1
  Angle/1 -> Add/1
  SP/1 -> Add/2
  PID Controller/1 -> Command/1

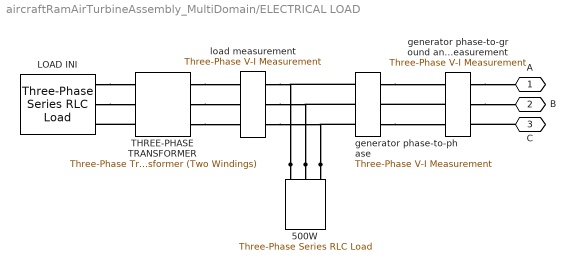
== system aircraftRamAirTurbineAssembly_MultiDomain/ELECTRICAL LOAD ==
  500W : powerlib/Elements/Three-Phase Series RLC Load  LConnTagsString=A|B|C  Configuration=Y (grounded)  NominalVoltage=200  NominalFrequency=400  ActivePower=500  InductivePower=0  CapacitivePower=0  Measurements=None  LoadType=constant Z
  LOAD INI : powerlib/Elements/Three-Phase Series RLC Load  LConnTagsString=A|B|C  Configuration=Y (grounded)  NominalVoltage=200  NominalFrequency=400  ActivePower=3e3  InductivePower=0  CapacitivePower=0  Measurements=None  LoadType=constant Z
  THREE-PHASE TRANSFORMER : powerlib/Elements/Three-Phase Transformer (Two Windings)  Winding1Connection=Delta (D1)  UNITS=pu  NominalPower=[ 25e3 , 400 ]  Winding1=[ 200 , 0.002 , 0.08 ]  Winding2Connection=Y  Winding2=[ 200 , 0.002 , 0.08 ]  SetSaturation=off  Rm=500  Lm=inf  Saturation=[ 0,0 ; 0.0024,1.2 ; 1.0,1.52 ]  Hysteresis=off  DataFile='hysteresis'  SetInitialFlux=off  InitialFluxes=[ 0.8 , -0.8 , 0.7 ]  Measurements=None  MoreParameters=off  BreakLoop=off  DataType=off  TransfoNumber=1
  "generator phase-to-ground and current measurement " : powerlib/Measurements/Three-Phase V-I Measurement  VoltageMeasurement=phase-to-ground  SetLabelV=on  LabelV=Vabc_SM  Vpu=on  VpuLL=off  CurrentMeasurement=yes  SetLabelI=on  LabelI=Iabc_SM  Ipu=off  Pbase=1e3  Vbase=200  OutputType=Magnitude  PhasorSimulation=off  PSBequivalent=0
  generator phase-to-phase : powerlib/Measurements/Three-Phase V-I Measurement  VoltageMeasurement=phase-to-phase  SetLabelV=on  LabelV=Vabc  Vpu=off  VpuLL=on  CurrentMeasurement=no  SetLabelI=on  LabelI=Iabc_SM  Ipu=off  Pbase=1e3  Vbase=200  OutputType=Magnitude  PhasorSimulation=off  PSBequivalent=0
  load measurement : powerlib/Measurements/Three-Phase V-I Measurement  VoltageMeasurement=phase-to-ground  SetLabelV=on  LabelV=Vabc_load  Vpu=off  VpuLL=off  CurrentMeasurement=yes  SetLabelI=on  LabelI=Iabc_load  Ipu=off  Pbase=100e6  Vbase=200  OutputType=Complex  PhasorSimulation=off  PSBequivalent=0
  A : PMIOPort  Port=1  Side=Right
  B : PMIOPort  Port=2  Side=Right
  C : PMIOPort  Port=3  Side=Right
  connections:
  500W/LConn1 -- load measurement/LConn1 -- generator phase-to-phase/RConn1
  500W/LConn2 -- load measurement/LConn2 -- generator phase-to-phase/RConn2
  500W/LConn3 -- load measurement/LConn3 -- generator phase-to-phase/RConn3
  generator phase-to-phase/LConn1 -- "generator phase-to-ground and current measurement "/RConn1
  "generator phase-to-ground and current measurement "/LConn1 -- A/RConn1
  "generator phase-to-ground and current measurement "/RConn2 -- generator phase-to-phase/LConn2
  THREE-PHASE TRANSFORMER/RConn3 -- LOAD INI/LConn3
  generator phase-to-phase/LConn3 -- "generator phase-to-ground and current measurement "/RConn3
  THREE-PHASE TRANSFORMER/LConn1 -- load measurement/RConn1
  LOAD INI/LConn2 -- THREE-PHASE TRANSFORMER/RConn2
  "generator phase-to-ground and current measurement "/LConn2 -- B/RConn1
  LOAD INI/LConn1 -- THREE-PHASE TRANSFORMER/RConn1
  THREE-PHASE TRANSFORMER/LConn2 -- load measurement/RConn2
  THREE-PHASE TRANSFORMER/LConn3 -- load measurement/RConn3
  C/RConn1 -- "generator phase-to-ground and current measurement "/LConn3

== system aircraftRamAirTurbineAssembly_MultiDomain/ELECTRICAL LOAD1 ==

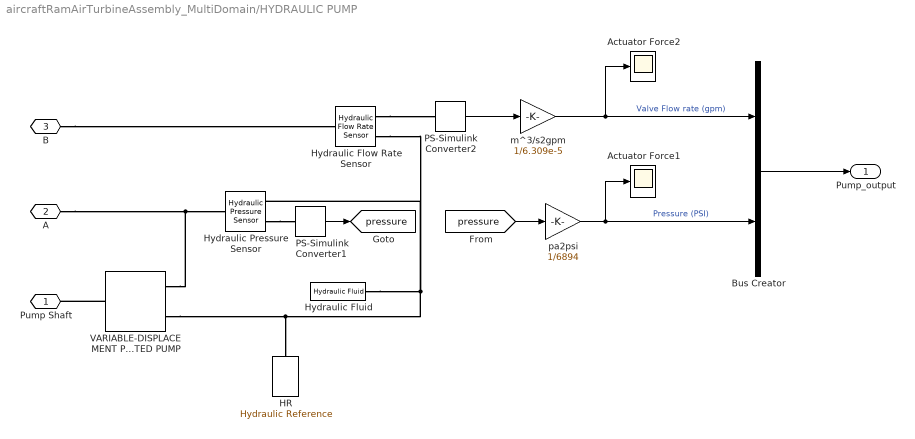
== system aircraftRamAirTurbineAssembly_MultiDomain/HYDRAULIC PUMP ==
  Actuator Force1 : Scope
      settings: TimeRange=5  YMin=1155.52  YMax=1155.75  SaveName=pump_pressure_psi
  Actuator Force2 : Scope
      settings: TimeRange=5  YMin=0.4  YMax=1.7  SaveName=pump_flow_gpm
  Bus Creator : BusCreator  Inputs=2
  HR : fl_lib/Hydraulic/Hydraulic Elements/Hydraulic Reference  Tag=Factory Generic  q_Log=off  LocalVarNames=|q  LocalVarDescs=|q  LocalVarLogging=[]
  Hydraulic Pressure Sensor : fl_lib/Hydraulic/Hydraulic Sensors/Hydraulic Pressure Sensor  Tag=Factory Generic  q_Log=off  p_Log=off  LocalVarNames=|q|p  LocalVarDescs=|q|p  LocalVarLogging=[]
  Hydraulic Flow Rate Sensor : fl_lib/Hydraulic/Hydraulic Sensors/Hydraulic Flow Rate Sensor  Tag=Factory Generic  q_Log=off  p_Log=off  LocalVarNames=|q|p  LocalVarDescs=|q|p  LocalVarLogging=[]
  Hydraulic Fluid : sh_lib/Hydraulic Utilities/Hydraulic Fluid  Tag=Factory Generic  DataSource=1  SelFluid=2  SysTemp=54 c  TrapAir=0.005  ViscDerFactor=1  LocalVarLogging=[]
  PS-Simulink Converter1 : nesl_utility/PS-Simulink Converter  PhysicalDomain=network_engine_domain  LeftPortType=input  RightPortType=output  SubClassName=ps_output  Unit=Pa  AffineConversion=off
  PS-Simulink Converter2 : nesl_utility/PS-Simulink Converter  PhysicalDomain=network_engine_domain  LeftPortType=input  RightPortType=output  SubClassName=ps_output  Unit=m^3/s  AffineConversion=off
  VARIABLE-DISPLACEMENT PRESSURE-COMPENSATED PUMP : sh_lib/Pumps and Motors/Variable-Displacement Pressure-Compensated Pump  D_max=4/8000 gal/rev  pr_set=1150 psi  pr_reg=50 psi  efficiency_vol=.97  efficiency_tot=0.95  pr_nominal=3000 psi  w_nominal=8000 rpm  visc_nominal=18 cSt  pump_delivery_Log=off  pr_drop_Log=off  leakage_flow_Log=off  torque_Log=off  ang_velocity_Log=off  displacement_Log=off  power_hyd_Log=off  LocalVarNames=|pump_delivery|pr_drop|leakage_flow|torque|ang_velocity|displacement|power_hyd  LocalVarDescs=|Pump delivery (m^3/s)|Pressure differential across the pump (Pa)|Leakage flow rate (m^3/s)|Driving shaft torque (N*m)|Driving shaft angular velocity (rad/s)|Pump displacement (m^3/rad)|Output flow power (W)  LocalVarLogging=[0 0 0 0 0 0 0]
  m^3/s2gpm : Gain  Gain=1/6.309e-5
  pa2psi : Gain  Gain=1/6894
  Pump Shaft : PMIOPort  Port=1  Side=Left
  A : PMIOPort  Port=2  Side=Right
  B : PMIOPort  Port=3  Side=Right
  Pump_output : Outport
  tag scope: pressure=global
  wires:
  PS-Simulink Converter2/1 -> m^3/s2gpm/1
  Bus Creator/1 -> Pump_output/1
  pa2psi/1 -> Bus Creator/2, Actuator Force1/1  "Pressure (PSI)"
  m^3/s2gpm/1 -> Bus Creator/1, Actuator Force2/1  "Valve Flow rate (gpm)"
  PS-Simulink Converter1/1 -> [pressure]
  [pressure] -> pa2psi/1
  connections:
  Hydraulic Pressure Sensor/RConn2 -- PS-Simulink Converter1/LConn1
  Hydraulic Flow Rate Sensor/RConn1 -- PS-Simulink Converter2/LConn1
  A/RConn1 -- VARIABLE-DISPLACEMENT PRESSURE-COMPENSATED PUMP/RConn1 -- Hydraulic Pressure Sensor/LConn1
  VARIABLE-DISPLACEMENT PRESSURE-COMPENSATED PUMP/RConn2 -- HR/LConn1 -- Hydraulic Pressure Sensor/RConn1 -- Hydraulic Flow Rate Sensor/RConn2 -- Hydraulic Fluid/RConn1
  B/RConn1 -- Hydraulic Flow Rate Sensor/LConn1
  VARIABLE-DISPLACEMENT PRESSURE-COMPENSATED PUMP/LConn1 -- Pump Shaft/RConn1

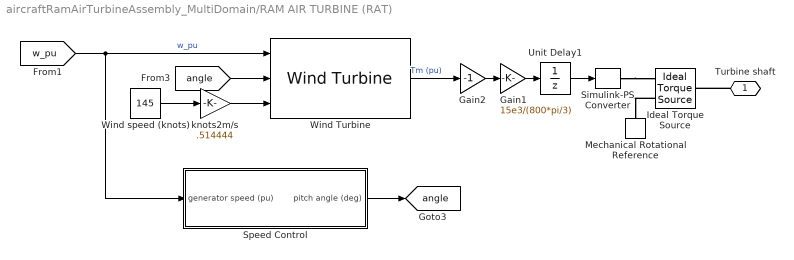
== system aircraftRamAirTurbineAssembly_MultiDomain/RAM AIR TURBINE (RAT) ==
  Gain1 : Gain  Gain=15e3/(800*pi/3)
  Gain2 : Gain  Gain=-1
  Ideal Torque Source : fl_lib/Mechanical/Mechanical Sources/Ideal Torque Source  w_Log=off  t_Log=off  LocalVarNames=|w|t  LocalVarDescs=|w|t  LocalVarLogging=[0 0]
  Mechanical Rotational Reference : fl_lib/Mechanical/Rotational Elements/Mechanical Rotational Reference  t_Log=off  LocalVarNames=|t  LocalVarDescs=|t  LocalVarLogging=0
  Simulink-PS Converter : nesl_utility/Simulink-PS Converter  PhysicalDomain=network_engine_domain  LeftPortType=input  RightPortType=output  SubClassName=ps_input  Unit=1  AffineConversion=off  InputFilterTimeConstant=.001  UdotUserProvided=0  SimscapeFilterOrder=1  InputFiltering=off
  Speed Control : Subsystem
  Unit Delay1 : UnitDelay  X0=15e3/(800*pi/3)  SampleTime=Ts
  Wind Turbine : DRlib/Wind Generation/Wind Turbine  Pnom=15e3  Pelec_base=1.5e4  wind_base=145*.514444  P_wind_base=1  speed_nom=1  pitch_angle=0  DisplayTurbChar=off  c1_c6="[0.51763          116          0.4            5           21     0.006795]"  cp_nom=0.48  lambda_nom=8.1
  Wind speed (knots) : Constant  Value=145
  knots2m/s : Gain  Gain=.514444
  Turbine shaft : PMIOPort  Port=1  Side=Left
  tag scope: angle=global
  wires:
  Speed Control/1(pitch angle (deg)) -> [angle]
  [angle] -> Wind Turbine/2
  Wind speed (knots)/1 -> knots2m/s/1
  Wind Turbine/1 -> Gain2/1  "Tm (pu)"
  [w_pu] -> Speed Control/1(generator speed (pu)), Wind Turbine/1  "w_pu"
  knots2m/s/1 -> Wind Turbine/3
  Gain1/1 -> Unit Delay1/1
  Gain2/1 -> Gain1/1
  Unit Delay1/1 -> Simulink-PS Converter/1
  connections:
  Ideal Torque Source/RConn2 -- Mechanical Rotational Reference/LConn1
  Simulink-PS Converter/RConn1 -- Ideal Torque Source/RConn1
  Turbine shaft/RConn1 -- Ideal Torque Source/LConn1

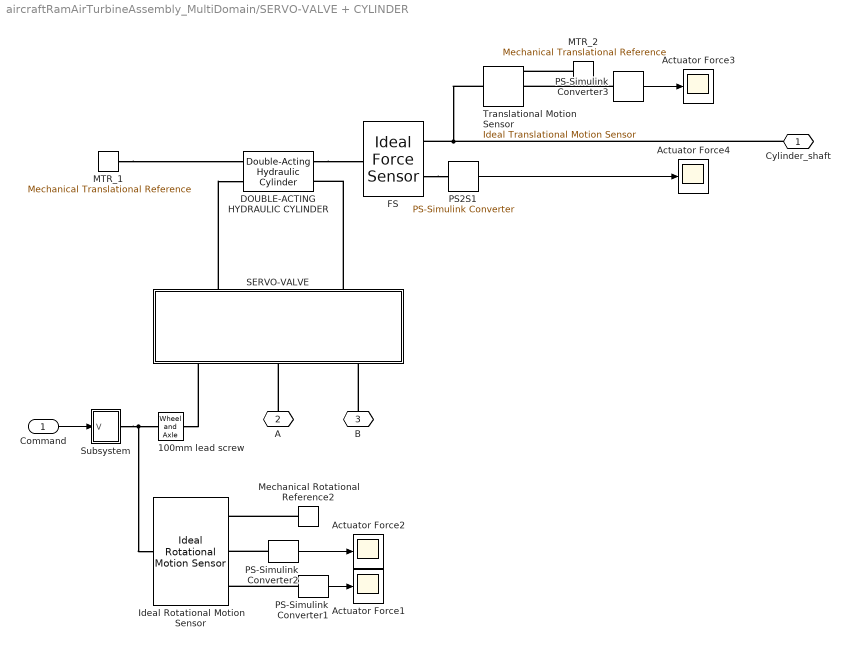
== system aircraftRamAirTurbineAssembly_MultiDomain/SERVO-VALVE + CYLINDER ==
  Command : Inport
  " Translational Motion Sensor" : fl_lib/Mechanical/Mechanical Sensors/Ideal Translational Motion Sensor  Tag=Factory Generic  offset=0 m  v_Log=off  f_Log=off  x_Log=off  LocalVarNames=|v|f|x  LocalVarDescs=|v|f|x  LocalVarLogging=[]
  100mm lead screw : fl_lib/Mechanical/Mechanisms/Wheel and Axle  R=100e-3/(2*pi) m  or=1  torque_A_Log=off  force_P_Log=off  ang_velocity_Log=off  velocity_Log=off  LocalVarNames=|torque_A|force_P|ang_velocity|velocity  LocalVarDescs=|Axle torque (N*m)|Periphery force (N)|Axle angular velocity (rad/s)|Periphery velocity (m/s)  LocalVarLogging=[0 0 0 0]
  Actuator Force{1..4} (4 alike) : Scope
      Actuator Force1 settings: TimeRange=5  YMin=0.00024  YMax=0.00038  SaveName=Aileron_EH_Force_DATA3
      Actuator Force2 settings: TimeRange=5  YMin=-0.05  YMax=0.05  SaveName=Aileron_EH_Force_DATA1
      Actuator Force3 settings: TimeRange=5  YMin=0.0004  YMax=0.0018  SaveName=Aileron_EH_Force_DATA9
      Actuator Force4 settings: TimeRange=5  YMin=0.0004  YMax=0.0018  SaveName=Aileron_EH_Force_DATA8
  DOUBLE-ACTING HYDRAULIC CYLINDER : sh_lib/Hydraulic Cylinders/Double-Acting Hydraulic Cylinder  Tag=Factory Generic  area_A=0.001 m^2  area_B=0.001 m^2  stroke=0.3 m  init_pos=0.15 m  dead_vol_A=1e-4 m^3  dead_vol_B=1e-4 m^3  init_pressure_A=0 Pa  init_pressure_B=0 Pa  k_sh=1.4  stiff=1e6 N/m  D=210 N/(m/s)  or=1  LocalVarLogging=[]
  FS : fl_lib/Mechanical/Mechanical Sensors/Ideal Force Sensor  Tag=Factory Generic  v_Log=off  f_Log=off  LocalVarNames=|v|f  LocalVarDescs=|v|f  LocalVarLogging=[]
  Ideal Rotational Motion Sensor : fl_lib/Mechanical/Mechanical Sensors/Ideal Rotational Motion Sensor  offset=0 rad  w_Log=off  t_Log=off  phi_Log=off  LocalVarNames=|w|t|phi  LocalVarDescs=|w|t|phi  LocalVarLogging=[0 0 0]
  MTR_1 : fl_lib/Mechanical/Translational Elements/Mechanical Translational Reference  Tag=Factory Generic  f_Log=off  LocalVarNames=|f  LocalVarDescs=|f  LocalVarLogging=[]
  MTR_2 : fl_lib/Mechanical/Translational Elements/Mechanical Translational Reference  Tag=Factory Generic  f_Log=off  LocalVarNames=|f  LocalVarDescs=|f  LocalVarLogging=[]
  Mechanical Rotational Reference2 : fl_lib/Mechanical/Rotational Elements/Mechanical Rotational Reference  t_Log=off  LocalVarNames=|t  LocalVarDescs=|t  LocalVarLogging=0
  PS-Simulink Converter1 : nesl_utility/PS-Simulink Converter  PhysicalDomain=network_engine_domain  LeftPortType=input  RightPortType=output  SubClassName=ps_output  Unit=1  AffineConversion=off
  PS-Simulink Converter2 : nesl_utility/PS-Simulink Converter  PhysicalDomain=network_engine_domain  LeftPortType=input  RightPortType=output  SubClassName=ps_output  Unit=1  AffineConversion=off
  PS-Simulink Converter3 : nesl_utility/PS-Simulink Converter  PhysicalDomain=network_engine_domain  LeftPortType=input  RightPortType=output  SubClassName=ps_output  Unit=1  AffineConversion=off
  PS2S1 : nesl_utility/PS-Simulink Converter  PhysicalDomain=network_engine_domain  LeftPortType=input  RightPortType=output  SubClassName=ps_output  Unit=1  AffineConversion=off
  SERVO-VALVE : Subsystem
      mask Display:
      | plot([198.418507352471;198.418507352471], [5.66910021007061;25.5109509453177])
      | plot([189.914857037365;206.922157667577], [25.5109509453177;25.5109509453177])
      | plot([240.936758928001;240.936758928001], [5.66910021007061;25.5109509453177])
      | plot([232.433108612895;249.440409243107], [25.5109509453177;25.5109509453177])
      | plot([240.936758928001;240.936758928001], [76.5328528359532;56.6910021007061])
      | plot([232.433108612895;249.440409243107], [56.6910021007061;56.6910021007061])
      | plot([198.418507352471;198.418507352471], [76.5328528359532;56.6910021007061])
      | plot([189.914857037365;206.922157667577], [56.6910021007061;56.6910021007061])
      | plot([99.2092536762357;99.2092536762357], [76.5328528359532;5.66910021007061])
      | plot([141.727505251765;141.727505251765], [76.5328528359532;5.66910021007061])
      | plot([170.073006302118;170.073006302118], [76.5328528359532;5.66910021007061])
      | plot([269.282259978354;269.282259978354], [76.5328528359532;5.66910021007061])
      | patch([99.2092536762357;93.5401534661651;104.878353886306;99.2092536762357], [76.5328528359532;53.8564519956708;53.8564519956708;76.5328528359532], [0;0;0])
      | plot([99.2092536762357;93.5401534661651;104.878353886306;99.2092536762357], [76.5328528359532;53.8564519956708;53.8564519956708;76.5328528359532])
      | patch([141.727505251765;136.058405041695;147.396605461836;141.727505251765], [5.66910021007061;28.3455010503531;28.3455010503531;5.66910021007061], [0;0;0])
      | plot([141.727505251765;136.058405041695;147.396605461836;141.727505251765], [5.66910021007061;28.3455010503531;28.3455010503531;5.66910021007061])
      | plot([297.627761028707;340.146012604237], [5.66910021007061;76.5328528359532])
      | plot([297.627761028707;340.146012604237], [76.5328528359532;5.66910021007061])
      | plot([70.8637526258826;368.49151365459;368.49151365459;70.8637526258826;70.8637526258826], [76.5328528359532;76.5328528359532;5.66910021007061;5.66910021007061;76.5328528359532])
      | patch([297.627761028707;303.296861238778;311.800511553884;297.627761028707], [5.66910021007061;25.5109509453177;19.8418507352471;5.66910021007061], [0;0;0])
      | plot([297.627761028707;303.296861238778;311.800511553884;297.627761028707], [5.66910021007061;25.5109509453177;19.8418507352471;5.66910021007061])
      | patch([297.627761028707;303.296861238778;311.800511553884;297.627761028707], [76.5328528359532;56.6910021007061;62.3601023107767;76.5328528359532], [0;0;0])
      | plot([297.627761028707;303.296861238778;311.800511553884;297.627761028707], [76.5328528359532;56.6910021007061;62.3601023107767;76.5328528359532])
      | plot([62.3601023107767;374.16061386466], [82.2019530460238;82.2019530460238])
      | plot([65.194652415812;376.995163969696], [0;0])
      | plot([70.8637526258826;0;0;70.8637526258826;70.8637526258826], [53.8564519956708;53.8564519956708;25.5109509453177;25.5109509453177;53.8564519956708])
      | plot([22.6764008402824;51.0219018906355], [53.8564519956708;25.5109509453177])
      | plot([14.1727505251765;53.8564519956708], [14.1727505251765;68.0292025208473])
      | patch([56.6910021007061;42.5182515755296;51.0219018906355;56.6910021007061], [73.6983027309179;62.3601023107767;56.6910021007061;73.6983027309179], [0;0;0])
      | plot([56.6910021007061;42.5182515755296;51.0219018906355;56.6910021007061], [73.6983027309179;62.3601023107767;56.6910021007061;73.6983027309179])
  Subsystem : Subsystem
  Cylinder_shaft : PMIOPort  Port=1  Side=Right
  A : PMIOPort  Port=2  Side=Left
  B : PMIOPort  Port=3  Side=Left
  wires:
  PS2S1/1 -> Actuator Force4/1
  PS-Simulink Converter3/1 -> Actuator Force3/1
  Command/1 -> Subsystem/1(V)
  PS-Simulink Converter1/1 -> Actuator Force1/1
  PS-Simulink Converter2/1 -> Actuator Force2/1
  connections:
  Subsystem/RConn1 -- 100mm lead screw/LConn1 -- Ideal Rotational Motion Sensor/LConn1
  100mm lead screw/RConn1 -- SERVO-VALVE/LConn1
  MTR_1/LConn1 -- DOUBLE-ACTING HYDRAULIC CYLINDER/LConn1
  SERVO-VALVE/RConn1 -- DOUBLE-ACTING HYDRAULIC CYLINDER/LConn2
  DOUBLE-ACTING HYDRAULIC CYLINDER/RConn1 -- FS/LConn1
  SERVO-VALVE/RConn2 -- DOUBLE-ACTING HYDRAULIC CYLINDER/RConn2
  FS/RConn2 -- PS2S1/LConn1
  MTR_2/LConn1 -- " Translational Motion Sensor"/RConn1
  PS-Simulink Converter3/LConn1 -- " Translational Motion Sensor"/RConn2
  A/RConn1 -- SERVO-VALVE/LConn2
  B/RConn1 -- SERVO-VALVE/LConn3
  Mechanical Rotational Reference2/LConn1 -- Ideal Rotational Motion Sensor/RConn1
  PS-Simulink Converter1/LConn1 -- Ideal Rotational Motion Sensor/RConn3
  PS-Simulink Converter2/LConn1 -- Ideal Rotational Motion Sensor/RConn2
  " Translational Motion Sensor"/LConn1 -- FS/RConn1 -- Cylinder_shaft/RConn1

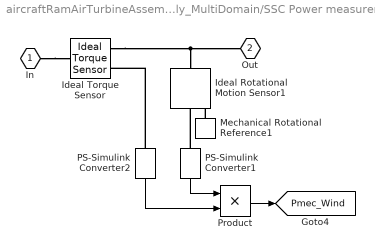
== system aircraftRamAirTurbineAssembly_MultiDomain/SSC Power measurement ==
  Ideal Rotational Motion Sensor1 : fl_lib/Mechanical/Mechanical Sensors/Ideal Rotational Motion Sensor  offset=0 deg  w_Log=off  t_Log=off  phi_Log=off  LocalVarNames=|w|t|phi  LocalVarDescs=|w|t|phi  LocalVarLogging=[0 0 0]
  Ideal Torque Sensor : fl_lib/Mechanical/Mechanical Sensors/Ideal Torque Sensor  w_Log=off  t_Log=off  LocalVarNames=|w|t  LocalVarDescs=|w|t  LocalVarLogging=[0 0]
  Mechanical Rotational Reference1 : fl_lib/Mechanical/Rotational Elements/Mechanical Rotational Reference  t_Log=off  LocalVarNames=|t  LocalVarDescs=|t  LocalVarLogging=0
  PS-Simulink Converter1 : nesl_utility/PS-Simulink Converter  PhysicalDomain=network_engine_domain  LeftPortType=input  RightPortType=output  SubClassName=ps_output  Unit=1  AffineConversion=off
  PS-Simulink Converter2 : nesl_utility/PS-Simulink Converter  PhysicalDomain=network_engine_domain  LeftPortType=input  RightPortType=output  SubClassName=ps_output  Unit=1  AffineConversion=off
  Product : Product  RndMeth=Zero
  In : PMIOPort  Port=1  Side=Left
  Out : PMIOPort  Port=2  Side=Right
  tag scope: Pmec_Wind=global
  wires:
  Product/1 -> [Pmec_Wind]
  PS-Simulink Converter2/1 -> Product/2
  PS-Simulink Converter1/1 -> Product/1
  connections:
  PS-Simulink Converter1/LConn1 -- Ideal Rotational Motion Sensor1/RConn2
  PS-Simulink Converter2/LConn1 -- Ideal Torque Sensor/RConn2
  Mechanical Rotational Reference1/LConn1 -- Ideal Rotational Motion Sensor1/RConn1
  Ideal Torque Sensor/RConn1 -- Out/RConn1 -- Ideal Rotational Motion Sensor1/LConn1
  In/RConn1 -- Ideal Torque Sensor/LConn1

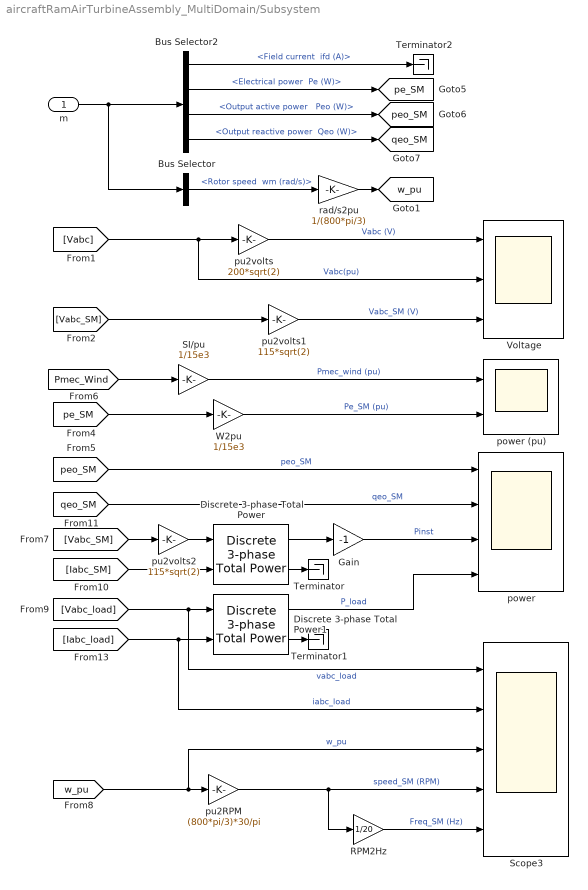
== system aircraftRamAirTurbineAssembly_MultiDomain/Subsystem ==
  m : Inport
  Bus Selector : BusSelector  OutputSignals="Mechanical.Rotor speed  wm (rad/s)"
  Bus Selector2 : BusSelector  OutputSignals="dq0 components.Field current  ifd (A),Mechanical.Electrical power  Pe (W),Output active power   Peo (W),Output reactive power  Qeo (W)"
  Discrete 3-phase Total Power : powerlib_extras/Discrete Measurements/Discrete 3-phase Total Power  Freq=400  Par_Vinit=[0 0]  Par_Iinit=[0 0]  Ts=Ts
  Discrete 3-phase Total Power1 : powerlib_extras/Discrete Measurements/Discrete 3-phase Total Power  Freq=400  Par_Vinit=[0 0]  Par_Iinit=[0 0]  Ts=Ts
  Gain : Gain  Gain=-1
  RPM2Hz : Gain  Gain=1/20
  SI/pu : Gain  Gain=1/15e3
  Scope3 : Scope  NumInputPorts=5
      settings: TimeRange=3  YMin=-200~-12.5~1~8000~400  YMax=200~12.5~1.175~9400~470  SaveName=results_2  SampleTime=Ts/100
  Terminator : Terminator
  Terminator1 : Terminator
  Terminator2 : Terminator
  Voltage : Scope  NumInputPorts=3
      settings: TimeRange=1  YMin=-300~-1~-175  YMax=300~1~175  SaveName=results_
  W2pu : Gain  Gain=1/15e3
  power : Scope  NumInputPorts=4
      settings: TimeRange=1  YMin=3390~59.5~-3490~2910  YMax=3500~66~-3370~3005  SaveName=results_3
  power (pu) : Scope  NumInputPorts=2
      settings: TimeRange=1  YMin=0.42811~0.23475  YMax=0.42831~0.23565  SaveName=results_1
  pu2RPM : Gain  Gain=(800*pi/3)*30/pi
  pu2volts : Gain  Gain=200*sqrt(2)
  pu2volts1 : Gain  Gain=115*sqrt(2)
  pu2volts2 : Gain  Gain=115*sqrt(2)
  rad/s2pu : Gain  Gain=1/(800*pi/3)
  tag scope: pe_SM=global, peo_SM=global, qeo_SM=global, w_pu=global
  wires:
  pu2volts/1 -> Voltage/1  "Vabc (V)"
  [Vabc] -> pu2volts/1, Voltage/2  "Vabc(pu)"
  [Pmec_Wind] -> SI/pu/1
  SI/pu/1 -> power (pu)/1  "Pmec_wind (pu)"
  pu2volts1/1 -> Voltage/3  "Vabc_SM (V)"
  [Vabc_SM] -> pu2volts1/1
  [qeo_SM] -> power/2  "qeo_SM"
  [Iabc_load] -> Discrete 3-phase Total Power1/2, Scope3/2  "iabc_load"
  [Vabc_load] -> Discrete 3-phase Total Power1/1, Scope3/1  "vabc_load"
  [peo_SM] -> power/1  "peo_SM"
  W2pu/1 -> power (pu)/2  "Pe_SM (pu)"
  [Vabc_SM] -> pu2volts2/1
  Discrete 3-phase Total Power1/2 -> Terminator1/1
  Discrete 3-phase Total Power/2 -> Terminator/1
  Discrete 3-phase Total Power/1 -> Gain/1
  [Iabc_SM] -> Discrete 3-phase Total Power/2
  pu2volts2/1 -> Discrete 3-phase Total Power/1
  [pe_SM] -> W2pu/1
  Gain/1 -> power/3  "Pinst"
  Discrete 3-phase Total Power1/1 -> power/4  "P_load"
  RPM2Hz/1 -> Scope3/5  "Freq_SM (Hz)"
  pu2RPM/1 -> RPM2Hz/1, Scope3/4  "speed_SM (RPM)"
  [w_pu] -> pu2RPM/1, Scope3/3  "w_pu"
  Bus Selector2/2 -> [pe_SM]  "<Electrical power  Pe (W)>"
  Bus Selector2/3 -> [peo_SM]  "<Output active power   Peo (W)>"
  Bus Selector2/4 -> [qeo_SM]  "<Output reactive power  Qeo (W)>"
  Bus Selector/1 -> rad/s2pu/1  "<Rotor speed  wm (rad/s)>"
  rad/s2pu/1 -> [w_pu]
  Bus Selector2/1 -> Terminator2/1  "<Field current  ifd (A)>"
  m/1 -> Bus Selector2/1, Bus Selector/1

== system aircraftRamAirTurbineAssembly_MultiDomain/Voltage Regulator ==
  SM Voltage Measurement : powerlib_extras/Discrete Measurements/Discrete 3-phase Sequence Analyzer  Freq=400  n=1  seq=Positive  Par_Init=[1 0]  Ts=Ts
  Terminator : Terminator
  Unit Delay1 : UnitDelay  X0=1  SampleTime=Ts
  Vmaxref_SM (pu) : Constant
  Voltage Regulator : Subsystem
  pu2volts : Gain  Gain=.57353
  Vf_exc (V) : Outport
  wires:
  Voltage Regulator/1(Vf_exc (pu)) -> pu2volts/1  "Vf_exc (pu)"
  [Vabc_SM] -> SM Voltage Measurement/1
  SM Voltage Measurement/2 -> Terminator/1
  SM Voltage Measurement/1 -> Unit Delay1/1
  pu2volts/1 -> Vf_exc (V)/1
  Vmaxref_SM (pu)/1 -> Voltage Regulator/1(Vmaxref_SM (pu))
  Unit Delay1/1 -> Voltage Regulator/2(Vmax_SM (pu))  "Vmax_SM (pu)"

== system aircraftRamAirTurbineAssembly_MultiDomain/RAM AIR TURBINE (RAT)/Speed Control ==
  generator speed (pu) : Inport
  Consigne : Constant
  Discrete PI Controller : powerlib_extras/Discrete  Control Blocks/Discrete PI Controller  Kp=60  Ki=100  Par_Limits=[90 0]  Init=0  Ts=Ts
  Sum : Sum  Inputs=|-+
  pitch angle (deg) : Outport
  wires:
  Sum/1 -> Discrete PI Controller/1  "erreur"
  Discrete PI Controller/1 -> pitch angle (deg)/1  "effort de commande"
  generator speed (pu)/1 -> Sum/2
  Consigne/1 -> Sum/1

== system aircraftRamAirTurbineAssembly_MultiDomain/SERVO-VALVE + CYLINDER/SERVO-VALVE ==
  Flapper-Nozzle : Subsystem
  Flapper/Armature : Subsystem
  Main Valve : Subsystem
  F : PMIOPort  Port=1  Side=Left
  P : PMIOPort  Port=2  Side=Left
  T : PMIOPort  Port=3  Side=Left
  A : PMIOPort  Port=4  Side=Right
  B : PMIOPort  Port=5  Side=Right
  connections:
  Flapper/Armature/RConn2 -- Flapper-Nozzle/LConn1
  Main Valve/LConn3 -- Flapper-Nozzle/LConn2 -- P/RConn1
  Flapper-Nozzle/RConn1 -- Main Valve/LConn1
  Flapper-Nozzle/RConn2 -- Main Valve/LConn2
  F/RConn1 -- Flapper/Armature/LConn1
  A/RConn1 -- Main Valve/RConn2
  B/RConn1 -- Main Valve/RConn3
  Main Valve/LConn4 -- T/RConn1
  Flapper/Armature/RConn1 -- Main Valve/RConn1

== system aircraftRamAirTurbineAssembly_MultiDomain/SERVO-VALVE + CYLINDER/Subsystem ==
  V : Inport
  Actuator Force : Scope  NumInputPorts=3
      settings: TimeRange=6  YMin=-0.25~-1.3~-0.08  YMax=0.15~-2.22045e-16~0  SaveName=Aileron_EH_Force_DATA4
  Actuator Force2 : Scope
      settings: TimeRange=10  YMin=-30000  YMax=40000  SaveName=Aileron_EH_Force_DATA5
  Bus Selector : BusSelector  OutputSignals=Speed wm (rad/s),Armature current ia (A),Electrical torque Te (n m)
  Controlled Voltage Source : powerlib/Electrical Sources/Controlled Voltage Source  Initialize=off  Source_Type=DC  Amplitude=0  Phase=0  Frequency=0  Measurements=None
  DC Machine : powerlib/Machines/DC Machine  PresetModel=No  MechanicalLoad=Mechanical rotational port  FieldType=Permanent magnet  ShowDetailedParameters=on  RLa="[ 4.8  1600e-6]"  RLf="[ 240  120]"  Laf=1.8  MachineConstant=Torque constant (N.m/A)  Ke=1.8  Kt=0.0637  J=2.5e-4  Bm=1e-1  Tf=0  w0=0  Ifinit=1  TsPowergui=0  TsBlock=-1
  S : PMIOPort  Port=1  Side=Right
  wires:
  V/1 -> Controlled Voltage Source/1, Actuator Force2/1
  DC Machine/1 -> Bus Selector/1
  Bus Selector/1 -> Actuator Force/1  "<Speed wm (rad/s)>"
  Bus Selector/2 -> Actuator Force/2  "<Armature current ia (A)>"
  Bus Selector/3 -> Actuator Force/3  "<Electrical torque Te (n m)>"
  connections:
  Controlled Voltage Source/RConn1 -- DC Machine/LConn2
  Controlled Voltage Source/LConn1 -- DC Machine/RConn1
  S/RConn1 -- DC Machine/LConn1

== system aircraftRamAirTurbineAssembly_MultiDomain/Voltage Regulator/Voltage Regulator ==
  Vmaxref_SM (pu) : Inport
  Vmax_SM (pu) : Inport  Port=2
  Discrete PI Controller : powerlib_extras/Discrete  Control Blocks/Discrete PI Controller  Kp=15  Ki=15  Par_Limits=[2.2 -2.2]  Init=0  Ts=Ts
  Sum : Sum  Inputs=|+-
  Vf_exc (pu) : Outport
  wires:
  Sum/1 -> Discrete PI Controller/1
  Vmaxref_SM (pu)/1 -> Sum/1
  Discrete PI Controller/1 -> Vf_exc (pu)/1  "Vf_exc (pu)"
  Vmax_SM (pu)/1 -> Sum/2
